simulink library "FF_Library"  (R2024b)
settings: Solver=VariableStepAuto  StartTime=0.0  StopTime=10.0  RelTol=1e-3
undefined symbols (not defined in the file or in its folder): Slope1, Slope2
libraries: simulink x60
(part 1 of 4)
Description:
  | Version log: V01
  | Date:  2026-3-12
  | author: Qiang Sui & F&F
settings Model: Creator=uiv70484  LastModifiedBy=uiv70484

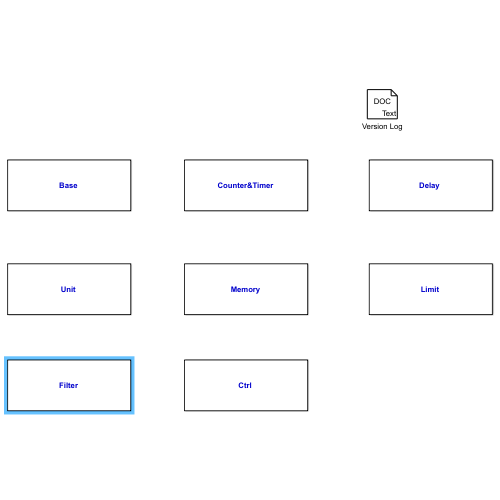
[thumbnail: Simulink's stored preview of the top-level diagram]
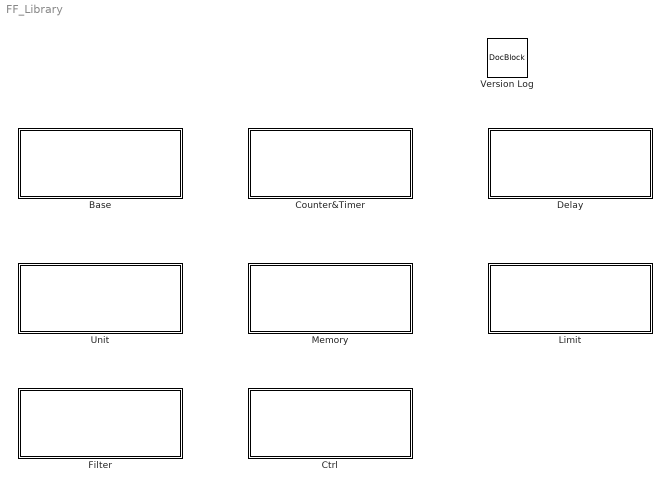
== system FF_Library ==
  Base : Subsystem
      mask Display:
      | color('blue');
      | name=get_param(gcb,'Name');
      | text(0.5,0.55,strcat('\fontsize{10}\bf',name),'HorizontalAlignment','center','VerticalAlignment','middle','texmode','on');
  Counter&Timer : Subsystem
      mask Display:
      | color('blue');
      | name=get_param(gcb,'Name');
      | text(0.5,0.55,strcat('\fontsize{10}\bf',name),'HorizontalAlignment','center','VerticalAlignment','middle','texmode','on');
  Ctrl : Subsystem
      mask Display:
      | color('blue');
      | name=get_param(gcb,'Name');
      | text(0.5,0.55,strcat('\fontsize{10}\bf',name),'HorizontalAlignment','center','VerticalAlignment','middle','texmode','on');
  Delay : Subsystem
      mask Display:
      | color('blue');
      | name=get_param(gcb,'Name');
      | text(0.5,0.55,strcat('\fontsize{10}\bf',name),'HorizontalAlignment','center','VerticalAlignment','middle','texmode','on');
  Filter : Subsystem
      mask Display:
      | color('blue');
      | name=get_param(gcb,'Name');
      | text(0.5,0.55,strcat('\fontsize{10}\bf',name),'HorizontalAlignment','center','VerticalAlignment','middle','texmode','on');
  Limit : Subsystem
      mask Display:
      | color('blue');
      | name=get_param(gcb,'Name');
      | text(0.5,0.55,strcat('\fontsize{10}\bf',name),'HorizontalAlignment','center','VerticalAlignment','middle','texmode','on');
  Memory : Subsystem
      mask Display:
      | color('blue');
      | name=get_param(gcb,'Name');
      | text(0.5,0.55,strcat('\fontsize{10}\bf',name),'HorizontalAlignment','center','VerticalAlignment','middle','texmode','on');
  Unit : Subsystem
      mask Display:
      | color('blue');
      | name=get_param(gcb,'Name');
      | text(0.5,0.55,strcat('\fontsize{10}\bf',name),'HorizontalAlignment','center','VerticalAlignment','middle','texmode','on');
  Version Log : simulink/Model-Wide Utilities/DocBlock  DocumentType=Text
      content=|
      | ************************Version log****************************************
      | Version log: V01
      | Date:  2026-3-12
      | author: Qiang Sui & F&F

== system FF_Library/Base ==
  DIV : Subsystem  mask(DIV){MinRange=1e-15}
      mask prompts: MinRange "smallest allowed value to divide by"
      mask help:
      | 除法模块：
      | 带有除0保护。
      mask Display:
      | port_label('input',1,'×');
      | port_label('input',2,'÷');
      | port_label('output',1,'');
  Decoder_16Bit : Subsystem  TreatAsAtomicUnit=on  mask(Decoder_16Bit){}
      mask help: Decoder_16Bit
      settings: RTWSystemCode=Inline
      mask Display: Constant=get_param(gcb,'Position');
  Decoder_8Bit : Subsystem  TreatAsAtomicUnit=on  mask(Decoder_8Bit){}
      mask help: Decoder_8Bit
      settings: RTWSystemCode=Inline
      mask Display: Constant=get_param(gcb,'Position');
  Encoder_16Bit : Subsystem  TreatAsAtomicUnit=on  mask(Encoder_16Bit){}
      mask help: Encoder_16Bit
      settings: RTWSystemCode=Inline
      mask Display: Constant=get_param(gcb,'Position');
  Encoder_8Bit : Subsystem  TreatAsAtomicUnit=on  mask(Encoder_8Bit){}
      mask help: Encoder_8Bit
      settings: RTWSystemCode=Inline
      mask Display: Constant=get_param(gcb,'Position');
  Flip_Unit16HighAndLowBit : Subsystem  mask(Flip_Unit16HighAndLowBit){}
      mask help:
      | Flip Unit16 Variable High And Low Bit
      | In:
      | In_Uint16  (Uint16 Variable)
      | Out :
      | Out_Uint16(Fliped Uint16 Variable)
      | Example:
      | In_Uint16=hex2dec('1234')
      | Out_Uint16=hex2dec('3412')
      mask Display: Constant=get_param(gcb,'Position');
  GetBit : Subsystem  TreatAsAtomicUnit=on  mask{maska=16}
      mask prompts: maska "bitAND with parameter"
      mask help:
      | Get Bit
      |
      | Implements Masked AND between the input and mask. If the result is grater than zero true is set to output - otherwise false.
      |
      | Block is useful for decoding bit-encoded data.
      |
      | Mask may not be a calibratable parameter.
      settings: RTWSystemCode=Inline
      mask Help:
      | Get Bit
      | 
      | Implements Masked AND between the input and mask. If the result is grater than zero true is set to output - otherwise false.
      | 
      | Block is useful for decoding bit-encoded data.
      | 
      | Mask may not be a calibratable parameter.
      mask Display:
      | Constant=get_param(gcb,'Position');
      | disp(['Input bitAND \n',maska]);
  Merge_Uint8ToUint16 : Subsystem  mask(Merge_Uint8ToUint16){}
      mask help:
      | Merge two Uint8 Variable To Uint16 Variable by bit
      | In:
      | In_Uint8_1  (Low 8 bit of Uint16 Variable)
      | In_Uint8_2  (High 8 bit of Uint16 Variable)
      | Out :
      | Out_Uint16(Uint16 Variable)
      | Example:
      | In_Uint8_1=hex2dec('12')
      | In_Uint8_2=hex2dec('34')
      | Out_Uint16=hex2dec('3412')
      mask Display: Constant=get_param(gcb,'Position');
  SetBit : Subsystem  TreatAsAtomicUnit=on  mask{maska=16}
      mask prompts: maska "Set to value"
      mask help:
      | Set Bit
      |
      | Sets the bit specified by value if the input is greater than zero.
      |
      | Block is useful for encoding bit-encoded data.
      |
      | "Set to value" may not be a calibratable parameter.
      settings: RTWSystemCode=Inline
      mask Help:
      | Set Bit
      | 
      | Sets the bit specified by value if the input is greater than zero.
      | 
      | Block is useful for encoding bit-encoded data.
      | 
      | "Set to value" may not be a calibratable parameter.
      mask Display: disp(['SetBit \n',maska]);

== system FF_Library/Counter&Timer ==
  COUNTDOWN_RE : Subsystem  mask(Output is true, if the number of block evaluations since the last reset is less than the initial number of block evaluations IV){}
      mask Display:
      | image(imread('CountDown_ASAM.tif','tif'),[0.29574 0.225 0.37895 0.55]);
      | disp('');
      | 
      | color('black');
      | port_label('input',1,'E');
      | port_label('input',2,'R');
      | port_label('input',3,'IV');
      | port_label('input',4,'x_in');
      | port_label('output',1,'y');
      | port_label('output',2,'x_out');
  COUNTUP_RE : Subsystem  mask(Counts up and gives out the number of block evaluations since the last reset.){}
      mask Display:
      | image(imread('Counter_ASAM.tif','tif'),[0.29574 0.225 0.37895 0.55]);
      | disp('');
      | 
      | color('black');
      | port_label('input',1,'E');
      | port_label('input',2,'R');
      | port_label('input',3,'IV');
      | port_label('input',4,'x_in');
      | port_label('output',1,'x_out');
  CounterCycle_SourceZero : Subsystem  mask(CounterCycle_SourceZero){CounterCycle=10}
      mask help:
      | CounterCycle_SourceZero is a discrete integrator for Integer variable.
      | This block can act as a source in model test,or as part of model.
      | CounterCycle:
      | The intergrator's CounterCycle.
      | Note:
      | The intergrator's initial value is 0.
      settings: AttributesFormatString=CounterCycle=%<CounterCycle>
      mask Display:
      | text(.1,.5,'\fontsize{10}\fontname{Courier New}\bfBMS\_ZeroBased','texmode','on');
      | plot([0.1 0.2 0.2 0.3 0.3 0.4 0.4 0.5  0.5 0.6 0.6 0.7 0.7 0.8 0.8  0.9 0.9 1],[0.1 0.1 0.22 0.22 0.35 0.35 0.1 0.1 0.22  0.22 0.35 0.35 0.1 0.1 0.22 0.22 0.35 0.35])
      | try
      |     set_param(gcb,'AttributesFormatString','CounterCycle=%<CounterCycle>');% get the value name
      | end
  TIMER_RE : Subsystem  mask(The block indicates true, if the initial time IV has not passed since the last reset of the block. Reset can only be performed, if the counter has run down to zero.){}
      mask Display:
      | image(imread('Timer_ASAM.tif','tif'),[0.29574 0.28 0.37895 0.44]);disp('');
      | disp('');
      | 
      | color('black');
      | port_label('input',1,'dT');
      | port_label('input',2,'E');
      | port_label('input',3,'R');
      | port_label('input',4,'IV');
      | port_label('input',5,'x_in');
      | port_label('output',1,'y');
      | port_label('output',2,'x_out');
  Timer : Subsystem  mask(Timer){TimerBaseFlag=ZeroBase}
      mask prompts: TimerBaseFlag "TimerBase"
      mask help:
      | 用于计时的模块：
      | En为1时开始计时，En变为0时暂停计时，当En再变为1时，再继续计时；
      | Reset为1时计时清零；
      | Max为最大计时时间，计时时间达到Max时，Flag=1；
      | TimeBase计时基准，ZeroBase代表从0开始计时，即En为1时计时为0，OneBase代表从1开始计时，即En为1时计时为一个步长。
      mask Display: image('StopWatch_Reset.GIF', [25,20,20,20,100,100]);

== system FF_Library/Ctrl ==
  note: PID
  note: INTEGRATORT
  INTEGRATORK_REL : Subsystem  mask(INTEGRATORK_REL){}
      mask help:
      | A time discrete integrator with gain K and limitation of the integrator value y
      | to the maximum MX and the minimum MN.
      settings: AttributesFormatString=V.10.2
      mask Help: eval('open(which([get_param(gcb,''MaskType''),''.html'']))');
      mask Display:
      | image(imread('Integratork_ASAM.tif','tif'),[0.24842 0.37778 0.37895 0.24444]);
      | disp('');
      | 
      | color('black');
      | port_label('input',1,'MX');
      | port_label('input',2,'MN');
      | port_label('input',3,'K');
      | port_label('input',4,'dT');
      | port_label('input',5,'u');
      | port_label('input',6,'E');
      | port_label('input',7,'R');
      | port_label('input',8,'IV');
      | port_label('input',9,'x_in');
      | port_label('output',1,'B_min');
      | port_label('output',2,'B_max');
      | port_label('output',3,'x_out');
  INTEGRATORT_REL : Subsystem  mask(INTEGRATORT_REL){}
      mask help: A time discrete integrator with gain 1/T and limitation of the integrator value y to the maximum MX and the minimum MN.
      settings: AttributesFormatString=V.10.2
      mask Help: eval('open(which([get_param(gcb,''MaskType''),''.html'']))');
      mask Display:
      | image(imread('Integratort_ASAM.tif','tif'),[0.24842 0.37778 0.37895 0.24444]);
      | disp('');
      | 
      | color('black');
      | port_label('input',1,'MX');
      | port_label('input',2,'MN');
      | port_label('input',3,'T');
      | port_label('input',4,'dT');
      | port_label('input',5,'u');
      | port_label('input',6,'E');
      | port_label('input',7,'R');
      | port_label('input',8,'IV');
      | port_label('input',9,'x_in');
      | port_label('output',1,'B_min');
      | port_label('output',2,'B_max');
      | port_label('output',3,'x_out');
  Integrator : Subsystem  Description=|
      | Ini:Enable to clear output value and memory;
      | X:Input;
      | dT:step time(s);
  PID : Subsystem  mask(PID){}
      mask help: U(k)=Kp*e(k)+Ki*Σe(k)+Kd*[e(k)-e(k-1)]
      mask Display: disp('PID');
  PID_Norm : Subsystem
      mask Display: disp('PID');

== system FF_Library/Delay ==
  note: TurnOnDelay
  note: TurnOffDelay
  TURNOFFDELAYSAMPLE : Subsystem  mask(TURNOFFDELAYSAMPLE){}
      mask help: A falling edge of the input signal u is delayed by n block evaluations (E).
      settings: AttributesFormatString=V.10.1
      mask Help: eval('open(which([get_param(gcb,''MaskType''),''.html'']))');
      mask Display:
      | image(imread('Turnoffdelaysample_ASAM.tif','tif'),[0.29574 0.225 0.37895 0.55]);
      | disp('');
      | 
      | color('black');
      | port_label('input',1,'n');
      | port_label('input',2,'u');
      | port_label('input',3,'R');
      | port_label('input',4,'x_in');
      | port_label('output',1,'y');
      | port_label('output',2,'x_out');
  TURNONDELAYSAMPLE : Subsystem  mask(TURNONDELAYSAMPLE){}
      mask help: TurnOnDelaySample: A rising edge of the input signal u is delayed by n block evaluations.
      mask Help: eval('open(which([get_param(gcb,''MaskType''),''.html'']))');
      mask Display:
      | image(imread('Turnondelaysample_ASAM.tif','tif'),[0.29574 0.225 0.37895 0.55]);
      | disp('');
      | 
      | color('black');
      | port_label('input',1,'n');
      | port_label('input',2,'u');
      | port_label('input',3,'R');
      | port_label('input',4,'x_in');
      | port_label('output',1,'y');
      | port_label('output',2,'x_out');
  TurnOffDeb : Subsystem  mask(TurnOffDeb){}
      mask help:
      | 下降沿Debounce：
      | 输入有下降沿的时候触发Debounce，延迟时间达到后才响应下降沿；输入有上升沿的时候立马响应上升沿。
      mask Display: image('TurnOffDelay_Timer.GIF', [15,5,10,5,100,100]);
  TurnOffDelay : Subsystem
      mask Display:
      | image(imread('Turnoffdelaytime_ASAM.tif','tif'),[0.29574 0.28 0.37895 0.44]);
      | disp('');
      | port_label('input',1,'X');
      | port_label('input',2,'Delay');
      | port_label('input',3,'dT');
      | port_label('input',4,'Ini');
      | port_label('output',1,'Y');
  TurnOnDeb : Subsystem  mask(TurnOnDeb){}
      mask help:
      | 上升沿Debounce：
      | 输入有上升沿的时候触发Debounce，延迟时间达到后才响应上升沿；输入有下降沿的时候立马响应下降沿。
      mask Display: image('TurnOnDelay_Timer.GIF', [15,5,10,5,100,100]);
  TurnOnDelay : Subsystem
      mask Display:
      | image(imread('Turnondelaytime_ASAM.tif','tif'),[0.29574 0.28 0.37895 0.44]);
      | disp('');
      | port_label('input',1,'X');
      | port_label('input',2,'Delay');
      | port_label('input',3,'dT');
      | port_label('input',4,'Ini');
      | port_label('output',1,'Y');

== system FF_Library/Filter ==
  note: Moving Average
  note: BandPass_Frequency
  note: LowPass_2阶
  note: HIGHPASST_RE
  note: LowPass_1阶
  note: if (R)
      | {
      | x1 = IV;
      | }
      | else if (E)
      | {
      | x1 = x1 + (TD*u - TD*x2 - dT*x1)/T;
      | }
      | x2 = u;
      | y = x1;
  note: if (R)
      | {
      | x1 = IV1;
      | x2 = IV2;
      | }
      | else if (E)
      | {
      | temp = x2[n-1];
      | temp1 = pow(T,2) + 2*D*T*dT;
      | x2[n] = x1[n-1];
      | x1[n] = x2 + [pow(dT, 2)*(u-x2)]
      | / temp1 + pow(T,2)*(x2 - temp) / temp1;
      | }
      | y = x1;
  BandPass_Frequency : Subsystem  Description=|
      | Ini:Enable to clear output value;
      | X:Input;
      | f_Up:Upper cut-off frequency(Hz);
      | f_Low:Lower cut-off frequency(Hz);
      | f_Low＜f_Up，both of them should be bigger than 0.01 Hz;
      | dT:step time(s);
      mask Display:
      | port_label('input', 1, 'lni');
      | port_label('input', 2, 'X');
      | port_label('input', 3, 'f_up');
      | port_label('input', 4, 'f_low');
      | port_label('input', 5, 'dT');
      | port_label('output', 1, 'y');
      | disp('BandPass');
  DIGITALLOWPASS_RE : Subsystem  mask(DIGITALLOWPASS_RE){}
      mask help: A discrete time first order lowpass.
      settings: AttributesFormatString=V.10.0
      mask Help: eval('open(which([get_param(gcb,''MaskType''),''.html'']))');
      mask Display:
      | image(imread('Lowpass_ASAM.tif','tif'),[0.29574 0.31667 0.37895 0.36667]);
      | disp('');
      | 
      | color('black');
      | port_label('input',1,'m');
      | port_label('input',2,'u');
      | port_label('input',3,'E');
      | port_label('input',4,'R');
      | port_label('input',5,'IV');
      | port_label('input',6,'x_in');
      | port_label('output',1,'y');
      | port_label('output',2,'x_out');
  HIGHPASST_RE : Subsystem
      mask Display:
      | image(imread('Highpass_ASAM.tif','tif'),[0.29574 0.37778 0.37895 0.24444]);
      | disp('');
  LOWPASSK_RE : Subsystem  mask(LOWPASSK_RE){}
      mask help: A discrete time 1. order lowpass filter with time constant 1/K.
      settings: AttributesFormatString=V.10.1
      mask Help: eval('open(which([get_param(gcb,''MaskType''),''.html'']))');
      mask Display:
      | image(imread('Lowpassk_ASAM.tif','tif'),[0.29574 0.34286 0.37895 0.31429]);
      | disp('');
      | 
      | color('black');
      | port_label('input',1,'K');
      | port_label('input',2,'dT');
      | port_label('input',3,'u');
      | port_label('input',4,'E');
      | port_label('input',5,'R');
      | port_label('input',6,'IV');
      | port_label('input',7,'x_in');
      | port_label('output',1,'y');
      | port_label('output',2,'x_out');
  LOWPASSSECORD_RE : Subsystem  mask(LOWPASSSECORD_RE){}
      mask help: A discrete time second order lowpass filter with time constant T and damping factor D (PT2).
      settings: AttributesFormatString=V.10.0
      mask Help: eval('open(which([get_param(gcb,''MaskType''),''.html'']))');
      mask Display:
      | image(imread('LowpassSecondOrder_ASAM.tif','tif'),[0.29574 0.39 0.37895 0.22]);
      | disp('');
      | 
      | color('black');
      | port_label('input',1,'T');
      | port_label('input',2,'D');
      | port_label('input',3,'dT');
      | port_label('input',4,'u');
      | port_label('input',5,'E');
      | port_label('input',6,'R');
      | port_label('input',7,'IV1');
      | port_label('input',8,'IV2');
      | port_label('input',9,'x1_in');
      | port_label('input',10,'x2_in');
      | port_label('output',1,'y');
      | port_label('output',2,'x1_out');
      | port_label('output',3,'x2_out');
  LOWPASST_RE : Subsystem  mask(LOWPASST_RE){}
      mask help: This block performs a first lowpass filter with T as time constant.
      settings: AttributesFormatString=V.11.0
      mask Help: eval('open(which([get_param(gcb,''MaskType''),''.html'']))');
      mask Display:
      | image(imread('Lowpasst_ASAM.tif','tif'),[0.29574 0.34286 0.37895 0.31429]);
      | disp('');
      | 
      | color('black');
      | port_label('input',1,'T');
      | port_label('input',2,'dT');
      | port_label('input',3,'u');
      | port_label('input',4,'E');
      | port_label('input',5,'R');
      | port_label('input',6,'IV');
      | port_label('input',7,'x_in');
      | port_label('output',1,'y');
      | port_label('output',2,'x_out');
  LowPass_Frequency : Subsystem  Description=|
      | Ini:Enable to clear output value;
      | X:Input;
      | f:Frequency(Hz)；
      | dT:step time(s);
      mask Display:
      | image(imread('LowPass_Frequency.jpg'),[0.29574 0.34286 0.37895 0.31429]);
      | port_label('input', 1, 'lni');
      | port_label('input', 2, 'X');
      | port_label('input', 3, 'f');
      | port_label('input', 4, 'dT');
      | port_label('output', 1, 'y');
  LowPass_K : Subsystem  Description=|
      | Suitable for high-frequency noise process.
      | Ini:Enable to clear output value;
      | X:Input;
      | K:LowPass factor;
      | dT:step time(s);
      | When K*dT=1, Y=X.
      mask Display:
      | port_label('input', 1, 'Ini');
      | port_label('input', 2, 'X');
      | port_label('input', 3, 'K');
      | port_label('input', 4, 'dT');
      | port_label('output', 1, 'Y');
      | image(imread('Lowpassk_ASAM.tif','tif'),[0.29574 0.34286 0.37895 0.31429]);
      | disp('');
  Moving_Average : Subsystem  mask(Moving Average){arraysize=3}
      mask prompts: arraysize "Buffer Size,value of buffer size must be larger than 0"
      mask help:
      | calculate the average of input value based on buffer size;
      | note: the dimention of input signal shall not be vector;
      mask Display:
      | image('Moving Average.GIF');
      | port_label('input', 1, 'u');
      | port_label('input', 2, 'R');
      | port_label('input', 3, 'IV');
      | text(0.4,0.1, ['buffer=',get_param(gcb,'arraysize')]);
  T-Filter : Subsystem  mask(T-Filter){}
      mask help: 该模块以T为时间常数执行一阶低通滤波器。
      mask Display: image('LowPassFilterT.GIF', [30,5,10,5,100,100]);

== system FF_Library/Limit ==
  note: DeadBand
  note: Hysteresis
  note: GradientLimiter
  ACCUMULATOR_REL : Subsystem  mask(ACCUMULATOR_REL){}
      mask help:
      | A time discrete integrator and limitation of the integrator value y
      | to the maximum MX and the minimum MN.
      settings: AttributesFormatString=V.10.2
      mask Help: eval('open(which([get_param(gcb,''MaskType''),''.html'']))');
      mask Display:
      | image(imread('Accumulator_ASAM.tif','tif'),[0.24842 0.34286 0.37895 0.31429]);
      | disp('');
      | 
      | color('black');
      | port_label('input',1,'MX');
      | port_label('input',2,'MN');
      | port_label('input',3,'u');
      | port_label('input',4,'E');
      | port_label('input',5,'R');
      | port_label('input',6,'IV');
      | port_label('input',7,'x_in');
      | port_label('output',1,'B_min');
      | port_label('output',2,'B_max');
      | port_label('output',3,'x_out');
  DIFFERENCELIMITER : Subsystem
      mask Display:
      | image(imread('DIFFERENCELIMITER_ASAM.tif','tif'),[0.24842 0.34286 0.37895 0.31429])
      | disp('');
  DeadBan_RE : Subsystem  mask(DeadBand){}
      mask help: Returns zero, if the input value is between UMIN and UMAX. Otherwise the output signal equals to the input signal reduced by the limits.
      mask Help: eval('open(which([get_param(gcb,''MaskType''),''.html'']))');
      mask Display:
      | image(imread('DeadBand.tif','tif'),[0.29574 0.17 0.37895 0.66])
      | disp('');
  DeadBand : Subsystem  mask(DeadBand){}
      mask help: 输入值 u 在 [MN, MX] 之间，输出 y 为 0；否则 y 为 u。
      mask Display: image('DeadBand.GIF', [10,10,10,10,100,100]);
  GRADIENTLIMITER : Subsystem
      mask Display:
      | image(imread('GRADIENTLIMITER_ASAM.tif','tif'),[0.24842 0.3625 0.37895 0.275])
      | disp('');
  Hysteresis : Subsystem  mask(Hysteresis){}
      mask help:
      | 如果输入值u＞RSP，输出y为1；直到输入值u＜LSP，输出y为0。
      | 初始输入u在 [LSP, RSP]之间，输出y为0。
      | 输入u、LSP、RSP需要有同样的数据类型。
      |
      | 输入：
      | LSP - 迟滞的left设定点
      | RSP - 迟滞的Right设定点
      | u      - 输入值
      | R     - Reset模块的Flag
      | RV   - Reset的值（boolean）
      |
      | 输出：
      | y      - 输出值（boolean）。当R为1，且u在 [LSP, RSP]之间，输出 y=RV。
      mask Display: image('Hysteresis.GIF', [20,5,10,5,100,100]);
  Hysteresis_Left : Subsystem
      mask help:
      | X>=Thd+HysDwn时Y输出为1，知道X下降到小于Thd时恢复为0；
      | 初始输入在Thd+HysDwn以下时输出y为0
      mask Display:
      | port_label('input', 1, 'X');
      | port_label('input', 2, 'Thd');
      | port_label('input', 3, 'HysDwn');
      | port_label('output', 1, 'Y');
      | disp('Hysteresis_Left');
  Hysteresis_Right : Subsystem
      mask help:
      | X>=Thd时Y输出为1，知道X下降到小于Thd-HysDwn时恢复为0；
      | 初始输入在Thd以下时输出y为0
      mask Display:
      | port_label('input', 1, 'X');
      | port_label('input', 2, 'Thd');
      | port_label('input', 3, 'HysDwn');
      | port_label('output', 1, 'Y');
      | disp('Hysteresis_Right');
  Limit : Subsystem  mask(Limit){}
      mask help:
      | 限制输入值u在[MN, MX]之间；
      | 所有的输入值必须是相同的数据类型。
      |
      | 输入：
      | MX - 允许的最大值
      | MN - 允许的最小值
      | u     - 输入值
      |
      | 输出：
      | y      -     受到限制的输出值
      | B_max - true，如果输入值u＞MX
      | B_min  - true，如果输入值u＜MN
      mask Display: image('Limit.GIF', [20,10,35,10,100,100]);
  Ramp : Subsystem  mask(Ramp){}
      mask help:
      | Limit rising and falling rates of signal.
      | dT(SampleTime) is the logic execution loop time.
      | RisingRamp is the positive gradient, when target value > base value, ramp step is RisingRamp*dT.
      | FailingRamp is the negtive gradient, when target value  < base value, ramp step is -1*FailingRamp*dT.
      mask Display: image('Ramp.GIF');

== system FF_Library/Memory ==
  note: FlipFlop
  note: SlideMemory
  note: Hold
  note: Edge
  note: Delta
  BooleanHold : Subsystem  mask(BooleanHold){True_Thd=0, False_Thd=0}
      mask help:
      | 若输入 u 由 0 跳变为 1，且经过“True_Thd”（uint16）周期后依然为 1，则输出 y = 1；
      | 若输入 u 由 1 跳变为 0，且经过“False_Thd”（uint16）周期后依然为 0，则输出 y = 0。
      |
      | 输入 u（boolean）；
      | 输出 y（boolean）；
      mask Display: disp('BooleanHold');
  DELTAONESTEP : Subsystem  mask(DELTAONESTEP){}
      mask help: Calculates the difference between the current and the last input value.
      settings: AttributesFormatString=V.10.1
      mask Help: eval('open(which([get_param(gcb,''MaskType''),''.html'']))');
      mask Display:
      | image(imread('Deltaonestep_ASAM.tif','tif'),[0.29574 0.225 0.37895 0.55]);
      | disp('');
      | 
      | color('black');
      | port_label('input',1,'u');
      | port_label('input',2,'R');
      | port_label('input',3,'IV');
      | port_label('input',4,'x_in');
      | port_label('output',1,'y');
      | port_label('output',2,'x_out');
  DIFFERENCEQUOTIENT : Subsystem  mask(DIFFERENCEQUOTIENT){}
      mask help: Calculates the rate of change of the input signal over time.
      settings: AttributesFormatString=V.10.1
      mask Help: eval('open(which([get_param(gcb,''MaskType''),''.html'']))');
      mask Display:
      | image(imread('Differencequotient_ASAM.tif','tif'),[0.29574 0.28 0.37895 0.44]);
      | disp('');
      | 
      | color('black');
      | port_label('input',1,'dT');
      | port_label('input',2,'u');
      | port_label('input',3,'R');
      | port_label('input',4,'IV');
      | port_label('input',5,'x_in');
      | port_label('output',1,'y');
      | port_label('output',2,'x_out');
  EDGEBI : Subsystem
      mask Display:
      | image(imread('Edgebi_ASAM.tif','tif'),[0.29574 0.225 0.37895 0.55]);
      | disp('');
  EDGEFALLING : Subsystem
      mask Display:
      | image(imread('Edgefalling_ASAM.tif','tif'),[0.29574 0.225 0.37895 0.55]);
      | disp('');
  EDGERAISING : Subsystem
      mask Display:
      | image(imread('Edgerising_ASAM.tif','tif'),[0.29574 0.225 0.37895 0.55]);
      | disp('');
  LoopHold : Subsystem  mask(LoopHold){LoopHold=0}
      mask prompts: LoopHold "Deb_Thd"
      mask help:
      | 输入u 初始值为“Init”的值。
      | 若输入 u 由 A 跳变为 B，且经过“Deb_Thd”（uint16）周期后依然为 B，则输出y = B；否则，y = A。
      |
      | 注：uint16 的数据范围要是不够，可以自行修改库模块中“LoopHold”的数据类型为 uint32。
      mask Display: disp('LoopHold');
  RSFlipFlop : Subsystem  mask(RSFlipFlop){}
      mask help:
      | RS触发器。第二个输入RST支配着第一个输入SET。
      |
      | 当RST为1，输出Q为0。当RST为0且SET为1，输出Q为1，并且在RST为0、SET由1变为0的基础上，输出Q保持上一值。
      mask Display:
      | port_label('input',1,'SET');
      | port_label('input',2,'RST');
      | port_label('output',1,'Q');
      | port_label('output',2,'~Q');
      | disp('RS FF');
  SAMPLEANDHOLD_RE : Subsystem  mask(SAMPLEANDHOLD_RE){}
      mask help: Sample and hold or just a simple memory block with enable and reset ports.
      settings: AttributesFormatString=V.10.0
      mask Help: eval('open(which([get_param(gcb,''MaskType''),''.html'']))');
      mask Display:
      | image(imread('Sampleandhold_ASAM.tif','tif'),[0.29574 0.28 0.37895 0.44]);
      | disp('');
      | 
      | color('black');
      | port_label('input',1,'u');
      | port_label('input',2,'E');
      | port_label('input',3,'R');
      | port_label('input',4,'IV');
      | port_label('input',5,'x_in');
      | port_label('output',1,'x_out');
  SRFlipFlop : Subsystem  mask(SRFlipFlop){}
      mask help:
      | SR触发器。第一个输入SET支配着第二个输入RST。
      |
      | 当SET为1，输出Q为1，并且在RST为0、SET由1变为0的基础上，输出Q保持上一值。当SET为0且RST为1，输出Q为0。
      mask Display:
      | port_label('input',1,'SET');
      | port_label('input',2,'RST');
      | port_label('output',1,'Q');
      | port_label('output',2,'~Q');
      | disp('SR FF');
  SlideMemory : Subsystem  Description=|
      | X:Input;
      | En:Enable condition（bool）；
      | num:Number of points in memory. It is equal to the size of A；
      | A:Ouput array；
      mask Display:
      | color('black');
      | port_label('input',1,'X');
      | port_label('input',2,'En');
      | port_label('input',3,'num');
      | port_label('output',1,'A');

== system FF_Library/Unit ==
  degps2radps : Subsystem
      mask Display: disp('degps2radps')
  g2mps2 : Subsystem
      mask Display: disp('g to mps2')
  mm to m2 : Subsystem
      mask Display: disp('mm to m')

== system FF_Library/Base/DIV ==
  In1 : Inport
  In2 : Inport  Port=2
  Constant2 : Constant  Value=abs(MinRange)  OutDataTypeStr=Inherit: Inherit via back propagation
  Constant3 : Constant  Value=-abs(MinRange)  OutDataTypeStr=Inherit: Inherit via back propagation
  Constant7 : Constant  Value=0  OutDataTypeStr=Inherit: Inherit via back propagation
  Divide1 : Product  Inputs=*/  SaturateOnIntegerOverflow=on
  Max2 : MinMax  Function=max  Inputs=2
  Min : MinMax  Inputs=2
  Relational Operator : RelationalOperator  OutDataTypeStr=boolean  RndMeth=Simplest  InputSameDT=off
  Switch : Switch  Criteria=u2 > Threshold  InputSameDT=off
  Out1 : Outport
  wires:
  Constant3/1 -> Min/2
  Min/1 -> Switch/3
  Constant2/1 -> Max2/2
  In1/1 -> Divide1/1
  Divide1/1 -> Out1/1
  Relational Operator/1 -> Switch/2
  Switch/1 -> Divide1/2
  Constant7/1 -> Relational Operator/2
  In2/1 -> Relational Operator/1, Max2/1, Min/1
  Max2/1 -> Switch/1

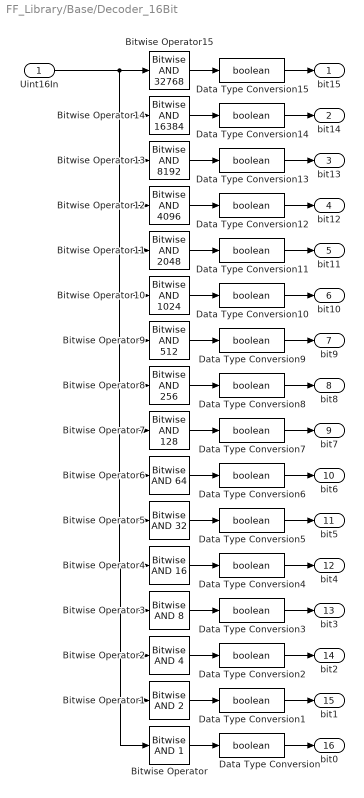
== system FF_Library/Base/Decoder_16Bit ==
  Uint16In : Inport  OutDataTypeStr=uint16
  Bitwise Operator : simulink/Logic and Bit Operations/Bitwise Operator  logicop=AND  UseBitMask=on  BitMask=1  BitMaskRealWorld=Stored Integer
  Bitwise Operator1 : simulink/Logic and Bit Operations/Bitwise Operator  logicop=AND  UseBitMask=on  BitMask=2  BitMaskRealWorld=Stored Integer
  Bitwise Operator10 : simulink/Logic and Bit Operations/Bitwise Operator  logicop=AND  UseBitMask=on  BitMask=1024  BitMaskRealWorld=Stored Integer
  Bitwise Operator11 : simulink/Logic and Bit Operations/Bitwise Operator  logicop=AND  UseBitMask=on  BitMask=2048  BitMaskRealWorld=Stored Integer
  Bitwise Operator12 : simulink/Logic and Bit Operations/Bitwise Operator  logicop=AND  UseBitMask=on  BitMask=4096  BitMaskRealWorld=Stored Integer
  Bitwise Operator13 : simulink/Logic and Bit Operations/Bitwise Operator  logicop=AND  UseBitMask=on  BitMask=8192  BitMaskRealWorld=Stored Integer
  Bitwise Operator14 : simulink/Logic and Bit Operations/Bitwise Operator  logicop=AND  UseBitMask=on  BitMask=16384  BitMaskRealWorld=Stored Integer
  Bitwise Operator15 : simulink/Logic and Bit Operations/Bitwise Operator  logicop=AND  UseBitMask=on  BitMask=32768  BitMaskRealWorld=Stored Integer
  Bitwise Operator2 : simulink/Logic and Bit Operations/Bitwise Operator  logicop=AND  UseBitMask=on  BitMask=4  BitMaskRealWorld=Stored Integer
  Bitwise Operator3 : simulink/Logic and Bit Operations/Bitwise Operator  logicop=AND  UseBitMask=on  BitMask=8  BitMaskRealWorld=Stored Integer
  Bitwise Operator4 : simulink/Logic and Bit Operations/Bitwise Operator  logicop=AND  UseBitMask=on  BitMask=16  BitMaskRealWorld=Stored Integer
  Bitwise Operator5 : simulink/Logic and Bit Operations/Bitwise Operator  logicop=AND  UseBitMask=on  BitMask=32  BitMaskRealWorld=Stored Integer
  Bitwise Operator6 : simulink/Logic and Bit Operations/Bitwise Operator  logicop=AND  UseBitMask=on  BitMask=64  BitMaskRealWorld=Stored Integer
  Bitwise Operator7 : simulink/Logic and Bit Operations/Bitwise Operator  logicop=AND  UseBitMask=on  BitMask=128  BitMaskRealWorld=Stored Integer
  Bitwise Operator8 : simulink/Logic and Bit Operations/Bitwise Operator  logicop=AND  UseBitMask=on  BitMask=256  BitMaskRealWorld=Stored Integer
  Bitwise Operator9 : simulink/Logic and Bit Operations/Bitwise Operator  logicop=AND  UseBitMask=on  BitMask=512  BitMaskRealWorld=Stored Integer
  Data Type Conversion{,1..15} (16 alike) : DataTypeConversion  OutDataTypeStr=boolean  SaturateOnIntegerOverflow=off  RndMeth=Floor
  bit15 : Outport  OutDataTypeStr=boolean  VectorParamsAs1DForOutWhenUnconnected=off
  bit14 : Outport  Port=2  OutDataTypeStr=boolean  VectorParamsAs1DForOutWhenUnconnected=off
  bit13 : Outport  Port=3  OutDataTypeStr=boolean  VectorParamsAs1DForOutWhenUnconnected=off
  bit12 : Outport  Port=4  OutDataTypeStr=boolean  VectorParamsAs1DForOutWhenUnconnected=off
  bit11 : Outport  Port=5  OutDataTypeStr=boolean  VectorParamsAs1DForOutWhenUnconnected=off
  bit10 : Outport  Port=6  OutDataTypeStr=boolean  VectorParamsAs1DForOutWhenUnconnected=off
  bit9 : Outport  Port=7  OutDataTypeStr=boolean  VectorParamsAs1DForOutWhenUnconnected=off
  bit8 : Outport  Port=8  OutDataTypeStr=boolean  VectorParamsAs1DForOutWhenUnconnected=off
  bit7 : Outport  Port=9  OutDataTypeStr=boolean  VectorParamsAs1DForOutWhenUnconnected=off
  bit6 : Outport  Port=10  OutDataTypeStr=boolean  VectorParamsAs1DForOutWhenUnconnected=off
  bit5 : Outport  Port=11  OutDataTypeStr=boolean  VectorParamsAs1DForOutWhenUnconnected=off
  bit4 : Outport  Port=12  OutDataTypeStr=boolean  VectorParamsAs1DForOutWhenUnconnected=off
  bit3 : Outport  Port=13  OutDataTypeStr=boolean  VectorParamsAs1DForOutWhenUnconnected=off
  bit2 : Outport  Port=14  OutDataTypeStr=boolean  VectorParamsAs1DForOutWhenUnconnected=off
  bit1 : Outport  Port=15  OutDataTypeStr=boolean  VectorParamsAs1DForOutWhenUnconnected=off
  bit0 : Outport  Port=16  OutDataTypeStr=boolean  VectorParamsAs1DForOutWhenUnconnected=off
  wires:
  Uint16In/1 -> Bitwise Operator12/1, Bitwise Operator6/1, Bitwise Operator/1, Bitwise Operator1/1, Bitwise Operator2/1, Bitwise Operator3/1, Bitwise Operator4/1, Bitwise Operator5/1, Bitwise Operator7/1, Bitwise Operator8/1, Bitwise Operator9/1, Bitwise Operator10/1, Bitwise Operator11/1, Bitwise Operator13/1, Bitwise Operator14/1, Bitwise Operator15/1
  Bitwise Operator/1 -> Data Type Conversion/1
  Data Type Conversion/1 -> bit0/1
  Bitwise Operator1/1 -> Data Type Conversion1/1
  Data Type Conversion1/1 -> bit1/1
  Bitwise Operator2/1 -> Data Type Conversion2/1
  Data Type Conversion2/1 -> bit2/1
  Bitwise Operator3/1 -> Data Type Conversion3/1
  Data Type Conversion3/1 -> bit3/1
  Bitwise Operator4/1 -> Data Type Conversion4/1
  Data Type Conversion4/1 -> bit4/1
  Bitwise Operator5/1 -> Data Type Conversion5/1
  Data Type Conversion5/1 -> bit5/1
  Bitwise Operator6/1 -> Data Type Conversion6/1
  Data Type Conversion6/1 -> bit6/1
  Bitwise Operator7/1 -> Data Type Conversion7/1
  Data Type Conversion7/1 -> bit7/1
  Bitwise Operator8/1 -> Data Type Conversion8/1
  Data Type Conversion8/1 -> bit8/1
  Bitwise Operator9/1 -> Data Type Conversion9/1
  Data Type Conversion9/1 -> bit9/1
  Bitwise Operator10/1 -> Data Type Conversion10/1
  Data Type Conversion10/1 -> bit10/1
  Bitwise Operator11/1 -> Data Type Conversion11/1
  Data Type Conversion11/1 -> bit11/1
  Bitwise Operator12/1 -> Data Type Conversion12/1
  Data Type Conversion12/1 -> bit12/1
  Bitwise Operator13/1 -> Data Type Conversion13/1
  Data Type Conversion13/1 -> bit13/1
  Bitwise Operator14/1 -> Data Type Conversion14/1
  Data Type Conversion14/1 -> bit14/1
  Bitwise Operator15/1 -> Data Type Conversion15/1
  Data Type Conversion15/1 -> bit15/1

== system FF_Library/Base/Decoder_8Bit ==
  Uint8In : Inport  OutDataTypeStr=uint8
  Bitwise Operator : simulink/Logic and Bit Operations/Bitwise Operator  logicop=AND  UseBitMask=on  BitMask=1  BitMaskRealWorld=Stored Integer
  Bitwise Operator1 : simulink/Logic and Bit Operations/Bitwise Operator  logicop=AND  UseBitMask=on  BitMask=2  BitMaskRealWorld=Stored Integer
  Bitwise Operator2 : simulink/Logic and Bit Operations/Bitwise Operator  logicop=AND  UseBitMask=on  BitMask=4  BitMaskRealWorld=Stored Integer
  Bitwise Operator3 : simulink/Logic and Bit Operations/Bitwise Operator  logicop=AND  UseBitMask=on  BitMask=8  BitMaskRealWorld=Stored Integer
  Bitwise Operator4 : simulink/Logic and Bit Operations/Bitwise Operator  logicop=AND  UseBitMask=on  BitMask=16  BitMaskRealWorld=Stored Integer
  Bitwise Operator5 : simulink/Logic and Bit Operations/Bitwise Operator  logicop=AND  UseBitMask=on  BitMask=32  BitMaskRealWorld=Stored Integer
  Bitwise Operator6 : simulink/Logic and Bit Operations/Bitwise Operator  logicop=AND  UseBitMask=on  BitMask=64  BitMaskRealWorld=Stored Integer
  Bitwise Operator7 : simulink/Logic and Bit Operations/Bitwise Operator  logicop=AND  UseBitMask=on  BitMask=128  BitMaskRealWorld=Stored Integer
  Data Type Conversion{,1..7} (8 alike) : DataTypeConversion  OutDataTypeStr=boolean  SaturateOnIntegerOverflow=off  RndMeth=Floor
  bit7 : Outport  OutDataTypeStr=boolean  VectorParamsAs1DForOutWhenUnconnected=off
  bit6 : Outport  Port=2  OutDataTypeStr=boolean  VectorParamsAs1DForOutWhenUnconnected=off
  bit5 : Outport  Port=3  OutDataTypeStr=boolean  VectorParamsAs1DForOutWhenUnconnected=off
  bit4 : Outport  Port=4  OutDataTypeStr=boolean  VectorParamsAs1DForOutWhenUnconnected=off
  bit3 : Outport  Port=5  OutDataTypeStr=boolean  VectorParamsAs1DForOutWhenUnconnected=off
  bit2 : Outport  Port=6  OutDataTypeStr=boolean  VectorParamsAs1DForOutWhenUnconnected=off
  bit1 : Outport  Port=7  OutDataTypeStr=boolean  VectorParamsAs1DForOutWhenUnconnected=off
  bit0 : Outport  Port=8  OutDataTypeStr=boolean  VectorParamsAs1DForOutWhenUnconnected=off
  wires:
  Data Type Conversion7/1 -> bit7/1
  Data Type Conversion6/1 -> bit6/1
  Data Type Conversion5/1 -> bit5/1
  Data Type Conversion4/1 -> bit4/1
  Data Type Conversion3/1 -> bit3/1
  Data Type Conversion2/1 -> bit2/1
  Data Type Conversion1/1 -> bit1/1
  Data Type Conversion/1 -> bit0/1
  Bitwise Operator6/1 -> Data Type Conversion6/1
  Bitwise Operator5/1 -> Data Type Conversion5/1
  Bitwise Operator2/1 -> Data Type Conversion2/1
  Bitwise Operator3/1 -> Data Type Conversion3/1
  Bitwise Operator4/1 -> Data Type Conversion4/1
  Bitwise Operator7/1 -> Data Type Conversion7/1
  Bitwise Operator1/1 -> Data Type Conversion1/1
  Uint8In/1 -> Bitwise Operator1/1, Bitwise Operator/1, Bitwise Operator2/1, Bitwise Operator3/1, Bitwise Operator4/1, Bitwise Operator5/1, Bitwise Operator6/1, Bitwise Operator7/1
  Bitwise Operator/1 -> Data Type Conversion/1

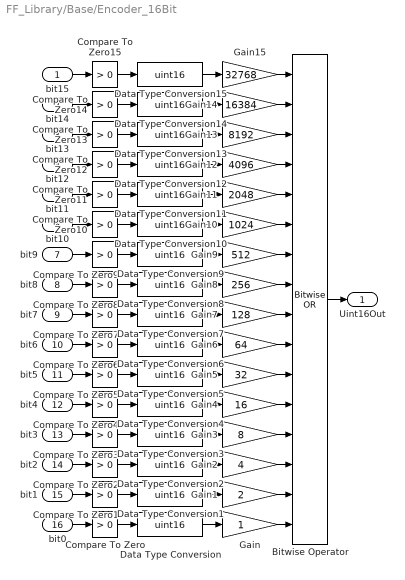
== system FF_Library/Base/Encoder_16Bit ==
  bit15 : Inport  OutDataTypeStr=boolean
  bit14 : Inport  Port=2  OutDataTypeStr=boolean
  bit13 : Inport  Port=3  OutDataTypeStr=boolean
  bit12 : Inport  Port=4  OutDataTypeStr=boolean
  bit11 : Inport  Port=5  OutDataTypeStr=boolean
  bit10 : Inport  Port=6  OutDataTypeStr=boolean
  bit9 : Inport  Port=7  OutDataTypeStr=boolean
  bit8 : Inport  Port=8  OutDataTypeStr=boolean
  bit7 : Inport  Port=9  OutDataTypeStr=boolean
  bit6 : Inport  Port=10  OutDataTypeStr=boolean
  bit5 : Inport  Port=11  OutDataTypeStr=boolean
  bit4 : Inport  Port=12  OutDataTypeStr=boolean
  bit3 : Inport  Port=13  OutDataTypeStr=boolean
  bit2 : Inport  Port=14  OutDataTypeStr=boolean
  bit1 : Inport  Port=15  OutDataTypeStr=boolean
  bit0 : Inport  Port=16  OutDataTypeStr=boolean
  Bitwise Operator : simulink/Logic and Bit Operations/Bitwise Operator  logicop=OR  UseBitMask=off  NumInputPorts=16  BitMask=bin2dec('11011001')  BitMaskRealWorld=Stored Integer
  Compare To Zero{,1..15} (16 alike) : simulink/Logic and Bit Operations/Compare To Zero  relop=>  OutDataTypeStr=boolean
  Data Type Conversion{,1..15} (16 alike) : DataTypeConversion  OutDataTypeStr=uint16  SaturateOnIntegerOverflow=off  RndMeth=Floor
  Gain : Gain  OutDataTypeStr=Inherit: Same as input
  Gain1 : Gain  Gain=2  OutDataTypeStr=Inherit: Same as input
  Gain10 : Gain  Gain=1024  OutDataTypeStr=Inherit: Same as input
  Gain11 : Gain  Gain=2048  OutDataTypeStr=Inherit: Same as input
  Gain12 : Gain  Gain=4096  OutDataTypeStr=Inherit: Same as input
  Gain13 : Gain  Gain=8192  OutDataTypeStr=Inherit: Same as input
  Gain14 : Gain  Gain=16384  OutDataTypeStr=Inherit: Same as input
  Gain15 : Gain  Gain=32768  OutDataTypeStr=Inherit: Same as input
  Gain2 : Gain  Gain=4  OutDataTypeStr=Inherit: Same as input
  Gain3 : Gain  Gain=8  OutDataTypeStr=Inherit: Same as input
  Gain4 : Gain  Gain=16  OutDataTypeStr=Inherit: Same as input
  Gain5 : Gain  Gain=32  OutDataTypeStr=Inherit: Same as input
  Gain6 : Gain  Gain=64  OutDataTypeStr=Inherit: Same as input
  Gain7 : Gain  Gain=128  OutDataTypeStr=Inherit: Same as input
  Gain8 : Gain  Gain=256  OutDataTypeStr=Inherit: Same as input
  Gain9 : Gain  Gain=512  OutDataTypeStr=Inherit: Same as input
  Uint16Out : Outport  OutDataTypeStr=uint16  VectorParamsAs1DForOutWhenUnconnected=off
  wires:
  Bitwise Operator/1 -> Uint16Out/1
  Compare To Zero5/1 -> Data Type Conversion5/1
  bit5/1 -> Compare To Zero5/1
  Data Type Conversion3/1 -> Gain3/1
  Data Type Conversion1/1 -> Gain1/1
  Data Type Conversion7/1 -> Gain7/1
  Data Type Conversion6/1 -> Gain6/1
  bit0/1 -> Compare To Zero/1
  Data Type Conversion5/1 -> Gain5/1
  Compare To Zero1/1 -> Data Type Conversion1/1
  Data Type Conversion2/1 -> Gain2/1
  bit6/1 -> Compare To Zero6/1
  Compare To Zero2/1 -> Data Type Conversion2/1
  bit4/1 -> Compare To Zero4/1
  bit1/1 -> Compare To Zero1/1
  Compare To Zero6/1 -> Data Type Conversion6/1
  bit3/1 -> Compare To Zero3/1
  Data Type Conversion/1 -> Gain/1
  Compare To Zero4/1 -> Data Type Conversion4/1
  bit2/1 -> Compare To Zero2/1
  Compare To Zero3/1 -> Data Type Conversion3/1
  Data Type Conversion4/1 -> Gain4/1
  Compare To Zero7/1 -> Data Type Conversion7/1
  bit7/1 -> Compare To Zero7/1
  Compare To Zero/1 -> Data Type Conversion/1
  bit8/1 -> Compare To Zero8/1
  Compare To Zero8/1 -> Data Type Conversion8/1
  Data Type Conversion8/1 -> Gain8/1
  Data Type Conversion9/1 -> Gain9/1
  Compare To Zero9/1 -> Data Type Conversion9/1
  bit9/1 -> Compare To Zero9/1
  bit10/1 -> Compare To Zero10/1
  Compare To Zero10/1 -> Data Type Conversion10/1
  Data Type Conversion10/1 -> Gain10/1
  Data Type Conversion11/1 -> Gain11/1
  Compare To Zero11/1 -> Data Type Conversion11/1
  bit11/1 -> Compare To Zero11/1
  bit12/1 -> Compare To Zero12/1
  Compare To Zero12/1 -> Data Type Conversion12/1
  Data Type Conversion12/1 -> Gain12/1
  Data Type Conversion13/1 -> Gain13/1
  Compare To Zero13/1 -> Data Type Conversion13/1
  bit13/1 -> Compare To Zero13/1
  bit14/1 -> Compare To Zero14/1
  Compare To Zero14/1 -> Data Type Conversion14/1
  Data Type Conversion14/1 -> Gain14/1
  Data Type Conversion15/1 -> Gain15/1
  Compare To Zero15/1 -> Data Type Conversion15/1
  bit15/1 -> Compare To Zero15/1
  Gain15/1 -> Bitwise Operator/1
  Gain14/1 -> Bitwise Operator/2
  Gain13/1 -> Bitwise Operator/3
  Gain12/1 -> Bitwise Operator/4
  Gain11/1 -> Bitwise Operator/5
  Gain10/1 -> Bitwise Operator/6
  Gain9/1 -> Bitwise Operator/7
  Gain8/1 -> Bitwise Operator/8
  Gain7/1 -> Bitwise Operator/9
  Gain6/1 -> Bitwise Operator/10
  Gain5/1 -> Bitwise Operator/11
  Gain4/1 -> Bitwise Operator/12
  Gain3/1 -> Bitwise Operator/13
  Gain2/1 -> Bitwise Operator/14
  Gain1/1 -> Bitwise Operator/15
  Gain/1 -> Bitwise Operator/16

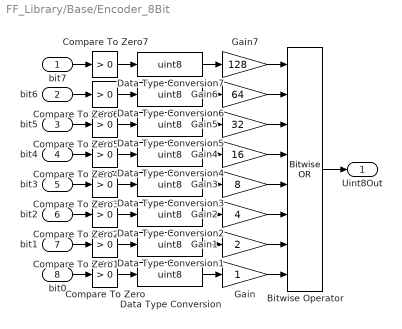
== system FF_Library/Base/Encoder_8Bit ==
  bit7 : Inport  OutDataTypeStr=boolean
  bit6 : Inport  Port=2  OutDataTypeStr=boolean
  bit5 : Inport  Port=3  OutDataTypeStr=boolean
  bit4 : Inport  Port=4  OutDataTypeStr=boolean
  bit3 : Inport  Port=5  OutDataTypeStr=boolean
  bit2 : Inport  Port=6  OutDataTypeStr=boolean
  bit1 : Inport  Port=7  OutDataTypeStr=boolean
  bit0 : Inport  Port=8  OutDataTypeStr=boolean
  Bitwise Operator : simulink/Logic and Bit Operations/Bitwise Operator  logicop=OR  UseBitMask=off  NumInputPorts=8  BitMask=bin2dec('11011001')  BitMaskRealWorld=Stored Integer
  Compare To Zero{,1..7} (8 alike) : simulink/Logic and Bit Operations/Compare To Zero  relop=>  OutDataTypeStr=boolean
  Data Type Conversion{,1..7} (8 alike) : DataTypeConversion  OutDataTypeStr=uint8  SaturateOnIntegerOverflow=off  RndMeth=Floor
  Gain : Gain  OutDataTypeStr=Inherit: Same as input
  Gain1 : Gain  Gain=2  OutDataTypeStr=Inherit: Same as input
  Gain2 : Gain  Gain=4  OutDataTypeStr=Inherit: Same as input
  Gain3 : Gain  Gain=8  OutDataTypeStr=Inherit: Same as input
  Gain4 : Gain  Gain=16  OutDataTypeStr=Inherit: Same as input
  Gain5 : Gain  Gain=32  OutDataTypeStr=Inherit: Same as input
  Gain6 : Gain  Gain=64  OutDataTypeStr=Inherit: Same as input
  Gain7 : Gain  Gain=128  OutDataTypeStr=Inherit: Same as input
  Uint8Out : Outport  OutDataTypeStr=uint8  VectorParamsAs1DForOutWhenUnconnected=off
  wires:
  Bitwise Operator/1 -> Uint8Out/1
  Gain/1 -> Bitwise Operator/8
  Gain1/1 -> Bitwise Operator/7
  Gain2/1 -> Bitwise Operator/6
  Gain3/1 -> Bitwise Operator/5
  Gain4/1 -> Bitwise Operator/4
  Gain5/1 -> Bitwise Operator/3
  Gain6/1 -> Bitwise Operator/2
  Gain7/1 -> Bitwise Operator/1
  Data Type Conversion/1 -> Gain/1
  Data Type Conversion1/1 -> Gain1/1
  Data Type Conversion2/1 -> Gain2/1
  Data Type Conversion3/1 -> Gain3/1
  Data Type Conversion4/1 -> Gain4/1
  Data Type Conversion5/1 -> Gain5/1
  Data Type Conversion6/1 -> Gain6/1
  Data Type Conversion7/1 -> Gain7/1
  bit0/1 -> Compare To Zero/1
  Compare To Zero/1 -> Data Type Conversion/1
  bit1/1 -> Compare To Zero1/1
  Compare To Zero1/1 -> Data Type Conversion1/1
  bit2/1 -> Compare To Zero2/1
  Compare To Zero2/1 -> Data Type Conversion2/1
  bit3/1 -> Compare To Zero3/1
  Compare To Zero3/1 -> Data Type Conversion3/1
  bit4/1 -> Compare To Zero4/1
  Compare To Zero4/1 -> Data Type Conversion4/1
  bit5/1 -> Compare To Zero5/1
  Compare To Zero5/1 -> Data Type Conversion5/1
  bit6/1 -> Compare To Zero6/1
  Compare To Zero6/1 -> Data Type Conversion6/1
  bit7/1 -> Compare To Zero7/1
  Compare To Zero7/1 -> Data Type Conversion7/1

== system FF_Library/Base/Flip_Unit16HighAndLowBit ==
  In_Uint16 : Inport
  Chart4 : Stateflow chart  TreatAsAtomicUnit=on
  Data Type Conversion : DataTypeConversion  OutDataTypeStr=uint16  SaturateOnIntegerOverflow=off  RndMeth=Floor
  Out_Uint16 : Outport  VectorParamsAs1DForOutWhenUnconnected=off
  wires:
  In_Uint16/1 -> Data Type Conversion/1
  Chart4/1(Out_Uint16) -> Out_Uint16/1
  Data Type Conversion/1 -> Chart4/1(In_Uint16)

== system FF_Library/Base/GetBit ==
  In1 : Inport
  BitwiseOperator5 : simulink/Logic and Bit Operations/Bitwise Operator  logicop=AND  UseBitMask=on  BitMask=eval(maska)  BitMaskRealWorld=Stored Integer
  Compare To Constant : simulink/Logic and Bit Operations/Compare To Constant  relop=>  const=0  OutDataTypeStr=boolean
  Data Type Conversion : DataTypeConversion  OutDataTypeStr=uint32  SaturateOnIntegerOverflow=off  RndMeth=Floor
  Out1 : Outport  VectorParamsAs1DForOutWhenUnconnected=off
  wires:
  In1/1 -> Data Type Conversion/1
  BitwiseOperator5/1 -> Compare To Constant/1
  Compare To Constant/1 -> Out1/1
  Data Type Conversion/1 -> BitwiseOperator5/1

== system FF_Library/Base/Merge_Uint8ToUint16 ==
  In_Uint8_1 : Inport
  In_Uint8_2 : Inport  Port=2
  Chart4 : Stateflow chart  TreatAsAtomicUnit=on
  Data Type Conversion : DataTypeConversion  OutDataTypeStr=uint8  SaturateOnIntegerOverflow=off  RndMeth=Floor
  Data Type Conversion1 : DataTypeConversion  OutDataTypeStr=uint8  SaturateOnIntegerOverflow=off  RndMeth=Floor
  Out_Uint16 : Outport  VectorParamsAs1DForOutWhenUnconnected=off
  wires:
  Chart4/1(Out_Uint16) -> Out_Uint16/1
  In_Uint8_1/1 -> Data Type Conversion/1
  In_Uint8_2/1 -> Data Type Conversion1/1
  Data Type Conversion/1 -> Chart4/1(In_Uint8_1)
  Data Type Conversion1/1 -> Chart4/2(In_Uint8_2)

== system FF_Library/Base/SetBit ==
  In1 : Inport
  Compare To Constant : simulink/Logic and Bit Operations/Compare To Constant  relop=>  const=0  OutDataTypeStr=boolean
  Data Type Conversion1 : DataTypeConversion  OutDataTypeStr=uint32  SaturateOnIntegerOverflow=off  RndMeth=Floor
  Gain : Gain  Gain=uint32(eval(maska))
  Out1 : Outport  VectorParamsAs1DForOutWhenUnconnected=off
  wires:
  Compare To Constant/1 -> Data Type Conversion1/1
  Gain/1 -> Out1/1
  In1/1 -> Compare To Constant/1
  Data Type Conversion1/1 -> Gain/1

== system FF_Library/Counter&Timer/COUNTDOWN_RE ==
  note: y
  note: x_out
  E : Inport
  R : Inport  Port=2
  IV : Inport  Port=3
  x_in : Inport  Port=4
  Functionality : Subsystem
  Rounding Function : Rounding  Operator=round
  x : Terminator
  y : Outport
  x_out : Outport  Port=2
  wires:
  IV/1 -> Rounding Function/1
  Functionality/1(y) -> y/1
  Functionality/2(x_out) -> x_out/1
  Rounding Function/1 -> Functionality/3(IV)
  Functionality/3(x) -> x/1
  E/1 -> Functionality/1(E)
  x_in/1 -> Functionality/4(x_in)
  R/1 -> Functionality/2(R)

== system FF_Library/Counter&Timer/COUNTUP_RE ==
  note: x_out
  note: y
  E : Inport
  R : Inport  Port=2
  IV : Inport  Port=3
  x_in : Inport  Port=4
  Functionality : Subsystem
  Rounding Function : Rounding  Operator=round
  y : Terminator
  x_out : Outport
  wires:
  Functionality/2(x_out) -> x_out/1
  Rounding Function/1 -> Functionality/3(IV)
  Functionality/1(y) -> y/1
  IV/1 -> Rounding Function/1
  R/1 -> Functionality/2(R)
  E/1 -> Functionality/1(E)
  x_in/1 -> Functionality/4(x_in)
